simulink model "EnablePort3"  (R2017b)
settings: Solver=FixedStepDiscrete  StartTime=0.0  StopTime=10.0  FixedStep=0.200000  RelTol=1e-3
settings Model: Creator=hbourbou  LastModifiedBy=hbourbou
settings DataIOCC: SaveFormat=StructureWithTime
settings OptimizationCC: LifeSpan=inf
settings DebuggingCC: SFExecutionAtInitializationDiag=none
settings HardwareCC: ProdBitPerSizeT=32  ProdBitPerPtrDiffT=32  ProdWordSize=32  ProdHWDeviceType=Specified
settings CodeAppCC: StateflowObjectComments=on

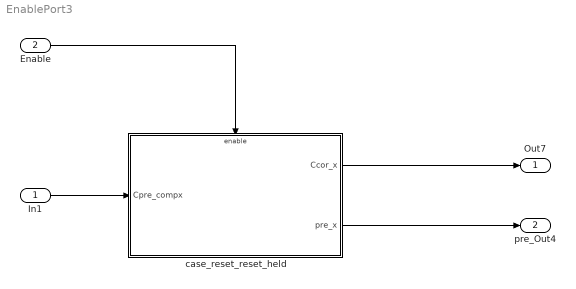
== system EnablePort3 ==
  In1 : Inport
  Enable : Inport  Port=2
  case_reset_reset_held : Subsystem  TreatAsAtomicUnit=on
  Out7 : Outport
  pre_Out4 : Outport  Port=2
  wires:
  In1/1 -> case_reset_reset_held/1(Cpre_compx)
  case_reset_reset_held/1(Ccor_x) -> Out7/1
  case_reset_reset_held/2(pre_x) -> pre_Out4/1
  Enable/1 -> case_reset_reset_held/Enable

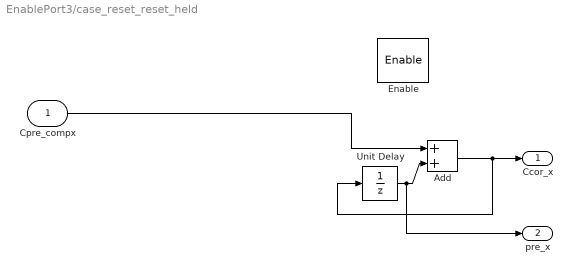
== system EnablePort3/case_reset_reset_held ==
  Cpre_compx : Inport  OutDataTypeStr=double  PortDimensions=[1]
  Enable : EnablePort  StatesWhenEnabling=reset
  Add : Sum
  Unit Delay : UnitDelay  SampleTime=-1.0000000000000000
  Ccor_x : Outport  OutputWhenDisabled=reset  InitialOutput=0
  pre_x : Outport  Port=2  InitialOutput=0
  wires:
  Cpre_compx/1 -> Add/1
  Add/1 -> Unit Delay/1, Ccor_x/1
  Unit Delay/1 -> pre_x/1, Add/2
